simulink model "lab4_dcm"  (R2021b)
settings: Solver=VariableStepAuto  StartTime=0.0  StopTime=10.0  RelTol=1e-3
values from neighbouring files (symbols this model uses):
  J = [Ixx 0 0; 0 Iyy 0; 0 0 Izz]    [euler_equation_tasks.m]    (also in lab5_task2.m)
  Jinv = inv(J)    [euler_equation_tasks.m]    (also in lab5_task2.m)
  w0 = [0.45 0.52 0.55]'    [euler_equation_tasks.m]    (also in lab5_task2.m = [C 0.1 0.1]')
undefined symbols (not defined in the file or in its folder): h_inertial
libraries: matrix_library x1
settings Model: Creator=samuz  LastModifiedBy=samuz

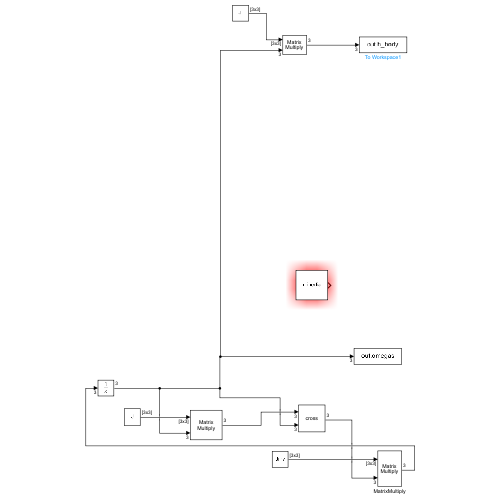
[thumbnail: Simulink's stored preview of the top-level diagram]
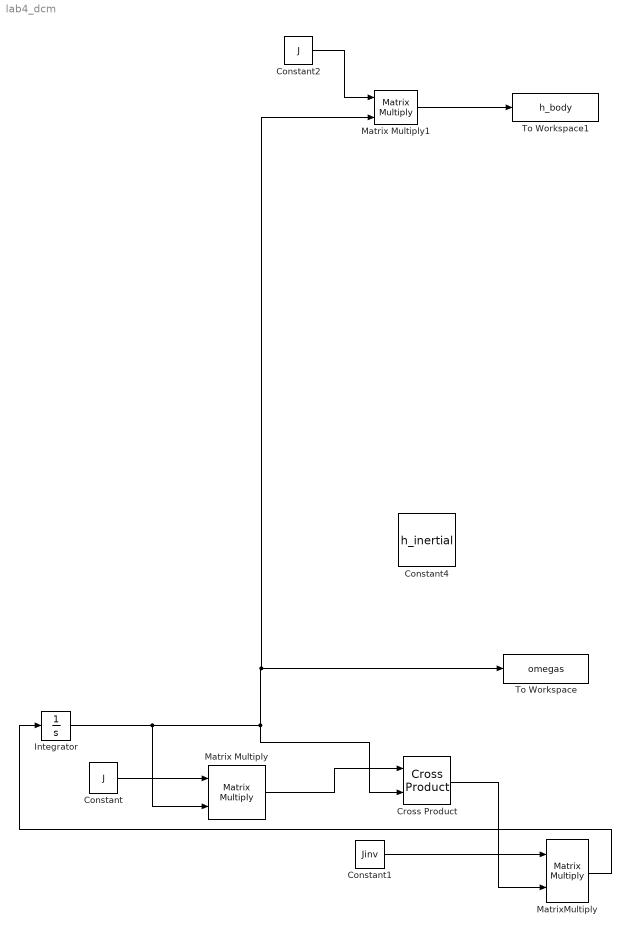
== system lab4_dcm ==
  Constant : Constant  Value=J
  Constant1 : Constant  Value=Jinv
  Constant2 : Constant  Value=J
  Constant4 : Constant  Value=h_inertial
  Cross Product : matrix_library/Cross Product
      settings: SourceProductBaseCode=SL
  Integrator : Integrator  InitialCondition=w0
  Matrix Multiply : Product  Multiplication=Matrix(*)
  Matrix Multiply1 : Product  Multiplication=Matrix(*)
  MatrixMultiply : Product  Multiplication=Matrix(*)
  To Workspace : ToWorkspace  VariableName=omegas  SampleTime=-1
  To Workspace1 : ToWorkspace  VariableName=h_body  SampleTime=-1
  wires:
  MatrixMultiply/1 -> Integrator/1
  Integrator/1 -> Matrix Multiply/2, Cross Product/2, Matrix Multiply1/2, To Workspace/1
  Cross Product/1 -> MatrixMultiply/2
  Constant1/1 -> MatrixMultiply/1
  Constant/1 -> Matrix Multiply/1
  Matrix Multiply/1 -> Cross Product/1
  Constant2/1 -> Matrix Multiply1/1
  Matrix Multiply1/1 -> To Workspace1/1
